simulink model "BoostConverter"  (R2020b)
settings: Solver=VariableStepAuto  StartTime=2  StopTime=2+(5*(1/Fs))  FixedStep=0.001  MaxStep=0.2  RelTol=1e-4  EnableMultiTasking=on
values from neighbouring files (symbols this model uses):
  C = (D*Iout)/(Vripple*Fs)    (= 0.0013)    [BoostConverter_data.m]    (also in BuckConverter_data.m = 4.7e-07; BuckConverter_data_deal.m = 2.5e-07)
  D = 1-(Vin/Vout)    (= 0.26)    [BoostConverter_data.m]    (also in BuckConverter_data.m = 0.2; BuckConverter_data_deal.m = 0.2)
  ESR_C = 13e-3    (= 0.013)    [BuckConverter_data.m]
  ESR_L = 56e-3    (= 0.056)    [BuckConverter_data.m]
  Fs = 40e3    (= 40000)    [BoostConverter_data.m]    (also in BuckConverter_data.m = 100000; BuckConverter_data_deal.m = 100000)
  L = (Vin*D)/(Iripple*Fs)    (= 0.00035594)    [BoostConverter_data.m]    (also in BuckConverter_data.m = 0.0012; BuckConverter_data_deal.m = 0.0012)
  Rout = 5000    [BoostConverter_data.m]    (also in BuckConverter_data.m = 1.5; BuckConverter_data_deal.m = 1.5)
  Vin = 3.7    [BoostConverter_data.m]    (also in BuckConverter_data.m = 15; BuckConverter_data_deal.m = 15)
libraries: powerlib x18
settings Model: Creator=Mateo C. Querol  LastModifiedBy=Mateo C. Querol
settings DataIOCC: LimitDataPoints=on  MaxDataPoints=10000  SaveOutput=off  ReturnWorkspaceOutputs=off
settings OptimizationCC: LifeSpan=inf
settings DebuggingCC: AllowSymbolicDim=off  SFUnexpectedBacktrackingDiag=warning  SFNoUnconditionalDefaultTransitionDiag=warning  SFExecutionAtInitializationDiag=none  ArithmeticOperatorsInVariantConditions=warning
settings SFSimCC: SimUseLocalCustomCode=off  CustomCodeUndefinedFunction=UseInterfaceOnly
settings RTWCC: RTWUseLocalCustomCode=off
settings CodeAppCC: StateflowObjectComments=on
settings GRTTargetCC: TargetLangStandard=C89/C90 (ANSI)
settings ConfigComp: CovMetricSettings=dw  CovSaveCumulativeToWorkspaceVar=on  CovSaveSingleToWorkspaceVar=on  CovExternalEMLEnable=off  CovSFcnEnable=off
settings SimscapeCC: SimscapeLogType=all  SimscapeLogDataHistory=10000

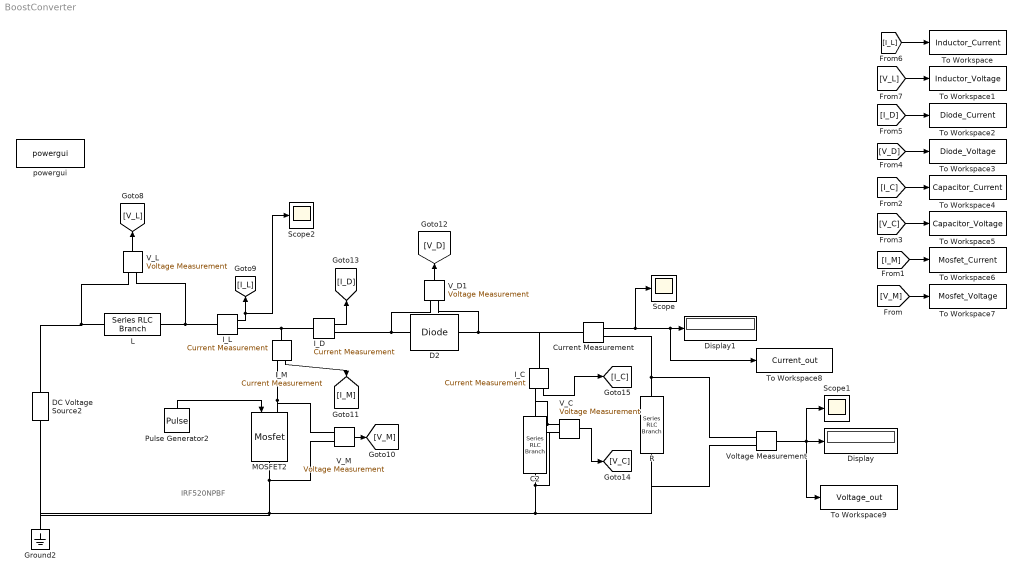
== system BoostConverter ==
  note: IRF520NPBF
  C2 : powerlib/Elements/Series RLC Branch  LConnTagsString=__new0  RConnTagsString=__new0  BranchType=C  Resistance=ESR_C  Inductance=1e-3  SetiL0=off  InitialCurrent=0  Capacitance=C  Setx0=off  InitialVoltage=0  Measurements=None
  Current Measurement : powerlib/Measurements/Current Measurement  PhasorSimulation=off  OutputType=Complex  PSBequivalent=0
  D2 : powerlib/Power Electronics/Diode  Ron=0.001  Lon=0  Vf=0  IC=0  UseSnubber=0  Rs=inf  Cs=inf  Measurements=off
  DC Voltage Source2 : powerlib/Electrical Sources/DC Voltage Source  Amplitude=Vin  Measurements=Voltage
  Display : Display
  Display1 : Display
  Ground2 : powerlib/Elements/Ground  LConnTagsString=a
  I_C : powerlib/Measurements/Current Measurement  PhasorSimulation=off  OutputType=Complex  PSBequivalent=0
  I_D : powerlib/Measurements/Current Measurement  PhasorSimulation=off  OutputType=Complex  PSBequivalent=0
  I_L : powerlib/Measurements/Current Measurement  PhasorSimulation=off  OutputType=Complex  PSBequivalent=0
  I_M : powerlib/Measurements/Current Measurement  PhasorSimulation=off  OutputType=Complex  PSBequivalent=0
  L : powerlib/Elements/Series RLC Branch  LConnTagsString=__new0  RConnTagsString=__new0  BranchType=L  Resistance=ESR_L  Inductance=L  SetiL0=off  InitialCurrent=0  Capacitance=1e-6  Setx0=off  InitialVoltage=0  Measurements=None
  MOSFET2 : powerlib/Power Electronics/Mosfet  Ron=0  Lon=0  Rd=0  Vfd=0  IC=0  Rs=inf  Cs=inf  Measurements=off
  Pulse Generator2 : DiscretePulseGenerator  PulseType=Time based  Amplitude=10  Period=1/Fs  PulseWidth=D*100
  R : powerlib/Elements/Series RLC Branch  LConnTagsString=__new0  RConnTagsString=__new0  BranchType=R  Resistance=Rout  Inductance=1e-3  SetiL0=off  InitialCurrent=0  Capacitance=1e-6  Setx0=off  InitialVoltage=0  Measurements=None
  Scope : Scope
  Scope1 : Scope
  Scope2 : Scope
  To Workspace : ToWorkspace  VariableName=Inductor_Current  SaveFormat=Timeseries  SampleTime=-1
      settings: Save2DSignal=2-D array (concatenate along first dimension)
  To Workspace1 : ToWorkspace  VariableName=Inductor_Voltage  SaveFormat=Timeseries  SampleTime=-1
      settings: Save2DSignal=2-D array (concatenate along first dimension)
  To Workspace2 : ToWorkspace  VariableName=Diode_Current  SaveFormat=Timeseries  SampleTime=-1
      settings: Save2DSignal=2-D array (concatenate along first dimension)
  To Workspace3 : ToWorkspace  VariableName=Diode_Voltage  SaveFormat=Timeseries  SampleTime=-1
      settings: Save2DSignal=2-D array (concatenate along first dimension)
  To Workspace4 : ToWorkspace  VariableName=Capacitor_Current  SaveFormat=Timeseries  SampleTime=-1
      settings: Save2DSignal=2-D array (concatenate along first dimension)
  To Workspace5 : ToWorkspace  VariableName=Capacitor_Voltage  SaveFormat=Timeseries  SampleTime=-1
      settings: Save2DSignal=2-D array (concatenate along first dimension)
  To Workspace6 : ToWorkspace  VariableName=Mosfet_Current  SaveFormat=Timeseries  SampleTime=-1
      settings: Save2DSignal=2-D array (concatenate along first dimension)
  To Workspace7 : ToWorkspace  VariableName=Mosfet_Voltage  SaveFormat=Timeseries  SampleTime=-1
      settings: Save2DSignal=2-D array (concatenate along first dimension)
  To Workspace8 : ToWorkspace  VariableName=Current_out  SampleTime=-1
      settings: Save2DSignal=2-D array (concatenate along first dimension)
  To Workspace9 : ToWorkspace  VariableName=Voltage_out  SampleTime=-1
      settings: Save2DSignal=2-D array (concatenate along first dimension)
  V_C : powerlib/Measurements/Voltage Measurement  PhasorSimulation=off  OutputType=Complex  PSBequivalent=0
  V_D1 : powerlib/Measurements/Voltage Measurement  PhasorSimulation=off  OutputType=Complex  PSBequivalent=0
  V_L : powerlib/Measurements/Voltage Measurement  PhasorSimulation=off  OutputType=Complex  PSBequivalent=0
  V_M : powerlib/Measurements/Voltage Measurement  PhasorSimulation=off  OutputType=Complex  PSBequivalent=0
  Voltage Measurement : powerlib/Measurements/Voltage Measurement  PhasorSimulation=off  OutputType=Complex  PSBequivalent=0
  powergui : powerlib/powergui  Priority=1  SimulationMode=Continuous  SampleTime=50e-6  frequency=60  Iterations=50  frequencyindice=0  Pbase=100e6  ErrMax=1e-4  UnitsV=kV  UnitsW=MW  buscounter=0  FunctionMessages=off  echomessages=off  EnableUseOfTLC=off  CurrentSourceSwitches=off  DisableSnubberDevices=off  DisableRonSwitches=off  DisableVfSwitches=off  DisplayEquations=off  AutomaticDiscreteSolvers=off  SolverType=Tustin/Backward Euler (TBE)  Interpol=off  ExternalGateDelay=off  methode=off  Ts=100  x0status=blocks  SPID=on  SwTol=0  HookPort=off  NonlinearTolerance=0  nMaxIteration=15  ContinueOnMaxIteration=off  RestoreLinks=warning  ResistiveCurrentMeasurement=off  Frange=[0:2:500]  Ylog=off  Xlog=on  ShowGrid=off  save=off  variable=ZData  structure=0  ZoomFFT=off  StartTime=0.0  cycles=1  DisplayStyle=1  fundamental=60  FreqAxis=off  MaxFrequency=1000  frequencyindicesteady=1  RmsSteady=1  display=off
  wires:
  [I_L] -> To Workspace/1
  [I_M] -> To Workspace6/1
  [V_D] -> To Workspace3/1
  [V_C] -> To Workspace5/1
  [I_C] -> To Workspace4/1
  [V_L] -> To Workspace1/1
  [V_M] -> To Workspace7/1
  [I_D] -> To Workspace2/1
  V_L/1 -> [V_L]
  I_L/1 -> Scope2/1, [I_L]
  V_M/1 -> [V_M]
  I_M/1 -> [I_M]
  Pulse Generator2/1 -> MOSFET2/1
  V_D1/1 -> [V_D]
  I_D/1 -> [I_D]
  V_C/1 -> [V_C]
  I_C/1 -> [I_C]
  Voltage Measurement/1 -> To Workspace9/1, Scope1/1, Display/1
  Current Measurement/1 -> Scope/1, To Workspace8/1, Display1/1
  connections:
  V_L/LConn1 -- DC Voltage Source2/RConn1 -- L/LConn1
  L/RConn1 -- I_L/LConn1 -- V_L/LConn2
  I_M/RConn1 -- V_M/LConn1 -- MOSFET2/LConn1
  I_L/RConn1 -- I_D/LConn1 -- I_M/LConn1
  C2/RConn1 -- Voltage Measurement/LConn2 -- R/RConn1 -- DC Voltage Source2/LConn1 -- Ground2/LConn1 -- V_M/LConn2 -- MOSFET2/RConn1 -- V_C/LConn2
  I_D/RConn1 -- D2/LConn1 -- V_D1/LConn1
  V_D1/LConn2 -- Current Measurement/LConn1 -- I_C/LConn1 -- D2/RConn1
  V_C/LConn1 -- C2/LConn1 -- I_C/RConn1
  R/LConn1 -- Current Measurement/RConn1 -- Voltage Measurement/LConn1
